simulink model "FIR_IIR_phase_response"  (R2016a)
settings: Solver=FixedStepDiscrete  SolverMode=SingleTasking  StartTime=0.0  StopTime=50  RelTol=1e-3
libraries: dspsrcs4 x3, dsparch4 x2
settings Model: Creator=mitia  LastModifiedBy=Chris
settings DataIOCC: LimitDataPoints=on  SaveFormat=Array  SignalLoggingSaveFormat=ModelDataLogs
settings OptimizationCC: BlockReduction=off  BooleanDataType=off  ExpressionDepthLimit=2147483647
settings DebuggingCC: SaveWithParameterizedLinksMsg=none  UnderspecifiedInitializationDetection=Classic  MergeDetectMultiDrivingBlocksExec=none  SignalResolutionControl=TryResolveAllWithWarning  MultiTaskDSMMsg=warning  MultiTaskCondExecSysMsg=none  StateNameClashWarn=warning  StrictBusMsg=None
settings HardwareCC: ProdBitPerPointer=32  ProdLargestAtomicFloat=None  ProdIntDivRoundTo=Undefined  ProdEndianess=Unspecified  ProdWordSize=32  ProdHWDeviceType=32-bit Generic  TargetUnknown=on
settings ModelReferenceCC: PropagateSignalLabelsOutOfModel=off
settings ConfigComp: CovModelRefEnable=Off

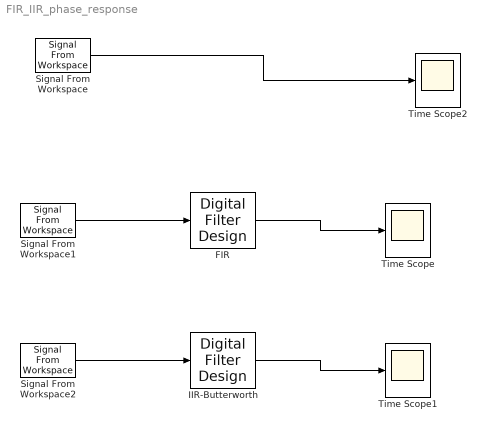
== system FIR_IIR_phase_response ==
  FIR : dsparch4/Digital Filter Design  mwdsp_browser_bugfix_var=off
  IIR-Butterworth : dsparch4/Digital Filter Design  mwdsp_browser_bugfix_var=off
  Signal From Workspace : dspsrcs4/Signal From Workspace  X=[ones(1,10) zeros(1,70)]  Ts=0.1  nsamps=1  OutputAfterFinalValue=Cyclic repetition  ignoreOrWarnInputAndFrameLengths=off  OutputFrames=on
  Signal From Workspace1 : dspsrcs4/Signal From Workspace  X=[ones(1,10) zeros(1,70)]  Ts=0.1  nsamps=1  OutputAfterFinalValue=Cyclic repetition  ignoreOrWarnInputAndFrameLengths=off  OutputFrames=on
  Signal From Workspace2 : dspsrcs4/Signal From Workspace  X=[ones(1,10) zeros(1,70)]  Ts=0.1  nsamps=1  OutputAfterFinalValue=Cyclic repetition  ignoreOrWarnInputAndFrameLengths=off  OutputFrames=on
  Time Scope : Scope
  Time Scope1 : Scope
  Time Scope2 : Scope
  wires:
  FIR/1 -> Time Scope/1
  Signal From Workspace2/1 -> IIR-Butterworth/1
  IIR-Butterworth/1 -> Time Scope1/1
  Signal From Workspace/1 -> Time Scope2/1
  Signal From Workspace1/1 -> FIR/1
